simulink model "Ex_1"  (R2020a)
settings: Solver=VariableStepAuto  StartTime=0.0  StopTime=0.05  RelTol=1e-3
settings Model: Creator=abhin  LastModifiedBy=abhin

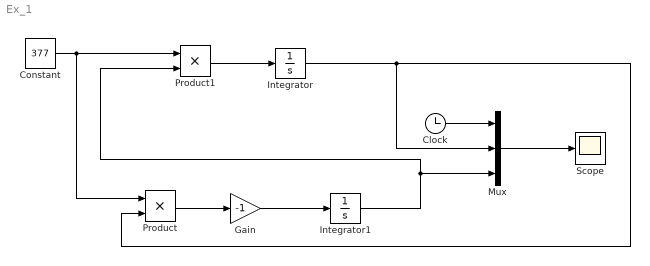
== system Ex_1 ==
  Clock : Clock
  Constant : Constant  Value=377
  Gain : Gain  Gain=-1
  Integrator : Integrator  InitialCondition=5
  Integrator1 : Integrator
  Mux : Mux  Inputs=3
  Product : Product
  Product1 : Product
  Scope : Scope
  wires:
  Constant/1 -> Product/1, Product1/1
  Product1/1 -> Integrator/1
  Product/1 -> Gain/1
  Gain/1 -> Integrator1/1
  Integrator1/1 -> Product1/2, Mux/3
  Integrator/1 -> Product/2, Mux/2
  Mux/1 -> Scope/1
  Clock/1 -> Mux/1
